simulink model "f8_VPP_demo_DER2"  (R2019b)
settings: Solver=VariableStepAuto  StartTime=0.0  StopTime=2  RelTol=1e-3
PreLoadFcn:
  | sr=0;ss=1;
InitFcn:
  | sr=0;ss=1;
undefined symbols (not defined in the file): Ion, Lithium
libraries: powerlib x185, powerlib_meascontrol x45, electricdrivelib x3, re_lib x3
(part 1 of 2)
settings Model: Creator=MAHMUD  LastModifiedBy=MAHMUD

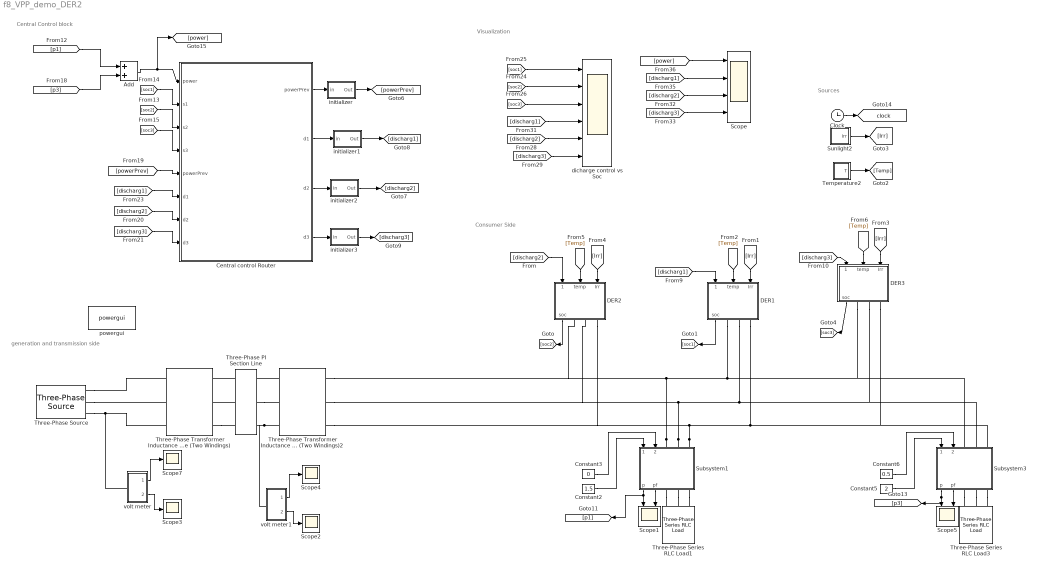
== system f8_VPP_demo_DER2 ==
  note: Consumer Side
  note: generation and transmission side
  note: Central Control block
  note: Visualization
  note: Sources
  Add : Sum  Inputs=2
  Central control Router : MATLAB Function  TreatAsAtomicUnit=on
  Clock : Clock
  Constant2 : Constant  Value=1.5
  Constant3 : Constant  Value=0
  Constant5 : Constant  Value=2
  Constant6 : Constant  Value=0.5
  DER1 : Subsystem
  DER2 : Subsystem
  DER3 : Subsystem
  Scope : Scope  NumInputPorts=4
  Scope1 : Scope  NumInputPorts=2
  Scope{2..4,7} (4 alike) : Scope
  Scope5 : Scope  NumInputPorts=2
  Subsystem1 : Subsystem
  Subsystem3 : Subsystem
  Sunlight2 : Subsystem
  Temperature2 : Subsystem
  Three-Phase PI Section Line : powerlib/Elements/Three-Phase PI Section Line  LConnTagsString=a|b|c  RConnTagsString=A|B|C  Frequency=50  Resistances=[ 0.01273 0.3864]  Inductances="[ 0.9337e-3  4.1264e-3]"  Capacitances=[12.74e-9 7.751e-9]  Length=100
      settings: SourceProductName=Simscape Electrical
  Three-Phase Series RLC Load1 : powerlib/Elements/Three-Phase Series RLC Load  LConnTagsString=A|B|C  Configuration=Y (grounded)  NominalVoltage=240  Vabc=[240 240 240]  Vabcp=[1e3 1e3 1e3]  NominalFrequency=50  UnbalancedPower=off  ActivePower=5e3  InductivePower=0  CapacitivePower=0  Pabc=[10e3 9e3 11e3]  QLabc=[100 90 110]  QCabc=[100 90 110]  Pabcp=[10e3 9e3 11e3]  QLabcp=[100 90 110]  QCabcp=[100 90 110]  Measurements=None  LoadType=constant PQ
      settings: SourceProductName=Simscape Electrical
  Three-Phase Series RLC Load3 : powerlib/Elements/Three-Phase Series RLC Load  LConnTagsString=A|B|C  Configuration=Y (grounded)  NominalVoltage=240  Vabc=[1e3 1e3 1e3]  Vabcp=[1e3 1e3 1e3]  NominalFrequency=50  UnbalancedPower=off  ActivePower=2e3  InductivePower=5e3  CapacitivePower=0  Pabc=[10e3 9e3 11e3]  QLabc=[100 90 110]  QCabc=[100 90 110]  Pabcp=[10e3 9e3 11e3]  QLabcp=[100 90 110]  QCabcp=[100 90 110]  Measurements=None  LoadType=constant PQ
      settings: SourceProductName=Simscape Electrical
  Three-Phase Source : powerlib/Electrical Sources/Three-Phase Source  InternalConnection=Yg  VoltagePhases=off  Voltage=14270  PhaseAngle=0  Voltage_phases=[25e3 25e3 25e3]/sqrt(3)  PhaseAngles_phases=[0 -120 +120]  Frequency=50  NonIdealSource=on  SpecifyImpedance=off  Resistance=0.8929  Inductance=0  ShortCircuitLevel=100e6  BaseVoltage=15000  XRratio=7  BusType=PQ  Pref=30e3  Qref=0  Prefabc=[10e3, 10e3, 10e3]  Qrefabc=[0, 0, 0]  Qmin=-inf  Qmax=inf
      settings: SourceProductName=Simscape Electrical
  Three-Phase Transformer Inductance Matrix Type (Two Windings) : powerlib/Elements/Three-Phase Transformer Inductance Matrix Type (Two Windings)  CoreType=Three-limb or five-limb core  Winding1Connection=Yg  Winding2Connection=Yg  AutoTransformer=off  Measurements=None  NominalPower=[100e3, 50]  VLLnom=[25000, 130000]  WindingResistances=[0.01, 0.01]  NoLoadIexcPos=2  NoLoadPlossPos=1000  ShortCircuitReactancePos=0.06  ShortCircuitReactancePosAuto=0.06  NoLoadIexcZero=100  NoLoadPlossZero=1500  ShortCircuitReactanceZero=0.03  ShortCircuitReactanceZeroAuto=0.03
      settings: SourceProductName=Simscape Electrical  SourceProductBaseCode=PS
  Three-Phase Transformer Inductance Matrix Type (Two Windings)2 : powerlib/Elements/Three-Phase Transformer Inductance Matrix Type (Two Windings)  CoreType=Three-limb or five-limb core  Winding1Connection=Yg  Winding2Connection=Yg  AutoTransformer=off  Measurements=None  NominalPower=[30e3, 50]  VLLnom=[12700, 240]  WindingResistances=[0.01, 0.01]  NoLoadIexcPos=4  NoLoadPlossPos=1000  ShortCircuitReactancePos=0.06  ShortCircuitReactancePosAuto=0.06  NoLoadIexcZero=100  NoLoadPlossZero=1500  ShortCircuitReactanceZero=0.03  ShortCircuitReactanceZeroAuto=0.03
      settings: SourceProductName=Simscape Electrical  SourceProductBaseCode=PS
  dicharge control vs Soc : Scope  NumInputPorts=6
  initializer : Subsystem
  initializer1 : Subsystem
  initializer2 : Subsystem
  initializer3 : Subsystem
  powergui : powerlib/powergui  Priority=1  SimulationMode=Continuous  SampleTime=50e-6  frequency=60  Iterations=50  frequencyindice=0  Pbase=100e6  ErrMax=1e-4  UnitsV=kV  UnitsW=MW  buscounter=0  FunctionMessages=off  echomessages=off  EnableUseOfTLC=off  CurrentSourceSwitches=off  DisableSnubberDevices=off  DisableRonSwitches=off  DisableVfSwitches=off  DisplayEquations=off  AutomaticDiscreteSolvers=off  SolverType=Tustin/Backward Euler (TBE)  Interpol=off  ExternalGateDelay=off  methode=off  Ts=100  x0status=blocks  SPID=on  SwTol=0  HookPort=off  NonlinearTolerance=1e-4  nMaxIteration=100  ContinueOnMaxIteration=off  RestoreLinks=warning  ResistiveCurrentMeasurement=off  Frange=[0:2:500]  Ylog=off  Xlog=on  ShowGrid=off  save=off  variable=ZData  structure=0  ZoomFFT=off  StartTime=0.0  cycles=1  DisplayStyle=1  fundamental=60  FreqAxis=off  MaxFrequency=1000  frequencyindicesteady=1  RmsSteady=1  display=off
      settings: SourceProductName=Simscape Electrical
  volt meter : Subsystem
  volt meter1 : Subsystem
  tag scope: clock=global
  wires:
  volt meter/1(Vsin) -> Scope7/1
  volt meter/2(Vrms) -> Scope3/1
  volt meter1/2(Vrms) -> Scope2/1
  volt meter1/1(Vsin) -> Scope4/1
  Subsystem1/1(p) -> [p1], Scope1/1
  Constant3/1 -> Subsystem1/2(start time)
  Constant6/1 -> Subsystem3/2(start time)
  Subsystem1/2(pf) -> Scope1/2
  Constant5/1 -> Subsystem3/1(stop time)
  Subsystem3/2(pf) -> Scope5/2
  Subsystem3/1(p) -> [p3], Scope5/1
  Constant2/1 -> Subsystem1/1(stop time)
  Temperature2/1(T) -> [Temp]
  Sunlight2/1(Irr) -> [Irr]
  [discharg2] -> DER2/1(discharging)
  [Temp] -> DER2/2(temp)
  [Irr] -> DER2/3(Irr)
  [Irr] -> DER1/3(Irr)
  [Temp] -> DER1/2(temp)
  [discharg1] -> DER1/1(discharging)
  [discharg3] -> DER3/1(discharging)
  [Temp] -> DER3/2(temp)
  [Irr] -> DER3/3(Irr)
  DER2/1(soc) -> [soc2]
  DER1/1(soc) -> [soc1]
  DER3/1(soc) -> [soc3]
  [p1] -> Add/1
  [p3] -> Add/2
  Central control Router/1(powerPrev) -> initializer/1(in)
  Central control Router/2(d1) -> initializer1/1(in)
  Central control Router/3(d2) -> initializer2/1(in)
  Central control Router/4(d3) -> initializer3/1(in)
  Add/1 -> [power], Central control Router/1(power)
  [soc3] -> Central control Router/4(s3)
  [soc1] -> Central control Router/2(s1)
  [soc2] -> Central control Router/3(s2)
  initializer3/1(Out) -> [discharg3]
  [powerPrev] -> Central control Router/5("powerPrev ")
  initializer/1(Out) -> [powerPrev]
  initializer2/1(Out) -> [discharg2]
  initializer1/1(Out) -> [discharg1]
  [discharg2] -> Central control Router/7("d2 ")
  [discharg3] -> Central control Router/8("d3 ")
  [discharg1] -> Central control Router/6("d1 ")
  Clock/1 -> [clock]
  [soc1] -> dicharge control vs Soc/1
  [soc2] -> dicharge control vs Soc/2
  [soc3] -> dicharge control vs Soc/3
  [power] -> Scope/1
  [discharg1] -> Scope/2
  [discharg2] -> Scope/3
  [discharg3] -> Scope/4
  [discharg1] -> dicharge control vs Soc/4
  [discharg2] -> dicharge control vs Soc/5
  [discharg3] -> dicharge control vs Soc/6
  connections:
  Three-Phase PI Section Line/RConn3 -- volt meter1/LConn1 -- Three-Phase Transformer Inductance Matrix Type (Two Windings)2/LConn3
  Three-Phase PI Section Line/RConn2 -- Three-Phase Transformer Inductance Matrix Type (Two Windings)2/LConn2
  Three-Phase PI Section Line/LConn1 -- Three-Phase Transformer Inductance Matrix Type (Two Windings)/RConn1
  Three-Phase Transformer Inductance Matrix Type (Two Windings)/RConn3 -- Three-Phase PI Section Line/LConn3
  Three-Phase PI Section Line/LConn2 -- Three-Phase Transformer Inductance Matrix Type (Two Windings)/RConn2
  Three-Phase Transformer Inductance Matrix Type (Two Windings)2/LConn1 -- Three-Phase PI Section Line/RConn1
  Three-Phase Source/RConn3 -- volt meter/LConn1 -- Three-Phase Transformer Inductance Matrix Type (Two Windings)/LConn3
  Three-Phase Source/RConn2 -- Three-Phase Transformer Inductance Matrix Type (Two Windings)/LConn2
  Three-Phase Source/RConn1 -- Three-Phase Transformer Inductance Matrix Type (Two Windings)/LConn1
  Subsystem1/LConn2 -- DER2/RConn2 -- Three-Phase Transformer Inductance Matrix Type (Two Windings)2/RConn2 -- Subsystem3/LConn2 -- DER3/RConn2 -- DER1/RConn2
  Subsystem1/LConn3 -- DER2/RConn3 -- Three-Phase Transformer Inductance Matrix Type (Two Windings)2/RConn3 -- Subsystem3/LConn3 -- DER3/RConn3 -- DER1/RConn3
  Subsystem1/LConn1 -- DER2/RConn1 -- Three-Phase Transformer Inductance Matrix Type (Two Windings)2/RConn1 -- Subsystem3/LConn1 -- DER3/RConn1 -- DER1/RConn1
  Subsystem1/RConn2 -- Three-Phase Series RLC Load1/LConn2
  Subsystem3/RConn3 -- Three-Phase Series RLC Load3/LConn3
  Subsystem3/RConn1 -- Three-Phase Series RLC Load3/LConn1
  Subsystem1/RConn1 -- Three-Phase Series RLC Load1/LConn1
  Subsystem1/RConn3 -- Three-Phase Series RLC Load1/LConn3
  Subsystem3/RConn2 -- Three-Phase Series RLC Load3/LConn2

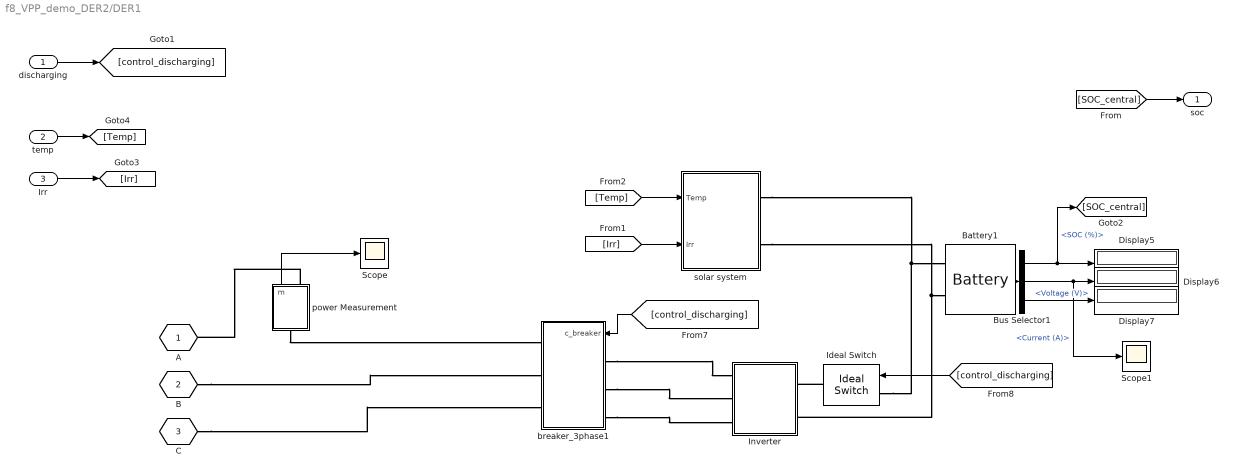
== system f8_VPP_demo_DER2/DER1 ==
  discharging : Inport
  temp : Inport  Port=2
  Irr : Inport  Port=3
  Battery1 : electricdrivelib/Extra Sources/Battery  BatType=Lithium-Ion  ShowTempParam=off  ThermalPreset=no  ShowAgeParam=off  NomV=100  NomQ=1000  SOC=5  Batt_Tr=0.1  PresetModel=on  MaxQ=1000  MinV=75  FullV=116.3987  Dis_rate=434.7826  R=0.001  Normal_OP=904.3478  expZone="[108.0386      49.13043]"  current=[6.5 13 32.5]  Units=Time  Tci=20  NomT=20  T2=-30  MaxQ2=4.8  FullV2=7.1  Normal_OP2=5.655  expZone2="[6.58           1]"  Rca=0.6  ti=2000  Dp=0  Neq0=0  Tsim=1e6  Ta1=25  Qeol=5.4*0.9  Reol=0.013333*1.2  Char_age=[2.3478, 3]  Dis_age=[2.3478, 10]  N1=1500  N2=10500  N3=1000  N4=1400  Ta2=45  N5=950
  Bus Selector1 : BusSelector  OutputSignals=SOC (%),Current (A),Voltage (V)
  Display5 : Display
  Display6 : Display
  Display7 : Display
  Ideal Switch : powerlib/Power Electronics/Ideal Switch  Ron=0.001  Lon=0  IC=0  Rs=1e5  Cs=inf  Measurements=off
      settings: SourceProductName=Simscape Electrical
  Inverter : Subsystem
  Scope : Scope
  Scope1 : Scope
  breaker_3phase1 : Subsystem
  power Measurement : Subsystem
  "solar system " : Subsystem
  A : PMIOPort  Tag=PMCPort  Side=Right
  B : PMIOPort  Tag=PMCPort  Port=2  Side=Right
  C : PMIOPort  Tag=PMCPort  Port=3  Side=Right
  soc : Outport
  wires:
  [SOC_central] -> soc/1
  [Temp] -> "solar system "/1(Temp)
  [Irr] -> "solar system "/2(Irr)
  temp/1 -> [Temp]
  Irr/1 -> [Irr]
  discharging/1 -> [control_discharging]
  [control_discharging] -> breaker_3phase1/1(c_breaker)
  [control_discharging] -> Ideal Switch/1
  power Measurement/1(m) -> Scope/1
  Bus Selector1/1 -> Display5/1, [SOC_central]  "<SOC (%)>"
  Battery1/1 -> Bus Selector1/1
  Bus Selector1/3 -> Display7/1  "<Voltage (V)>"
  Bus Selector1/2 -> Display6/1, Scope1/1  "<Current (A)>"
  connections:
  power Measurement/LConn1 -- breaker_3phase1/RConn1
  B/RConn1 -- breaker_3phase1/RConn2
  C/RConn1 -- breaker_3phase1/RConn3
  power Measurement/RConn1 -- A/RConn1
  breaker_3phase1/LConn2 -- Inverter/RConn2
  breaker_3phase1/LConn3 -- Inverter/RConn3
  breaker_3phase1/LConn1 -- Inverter/RConn1
  Ideal Switch/RConn1 -- Inverter/LConn1
  Battery1/LConn2 -- Inverter/LConn2 -- "solar system "/RConn2
  "solar system "/RConn1 -- Ideal Switch/LConn1 -- Battery1/LConn1

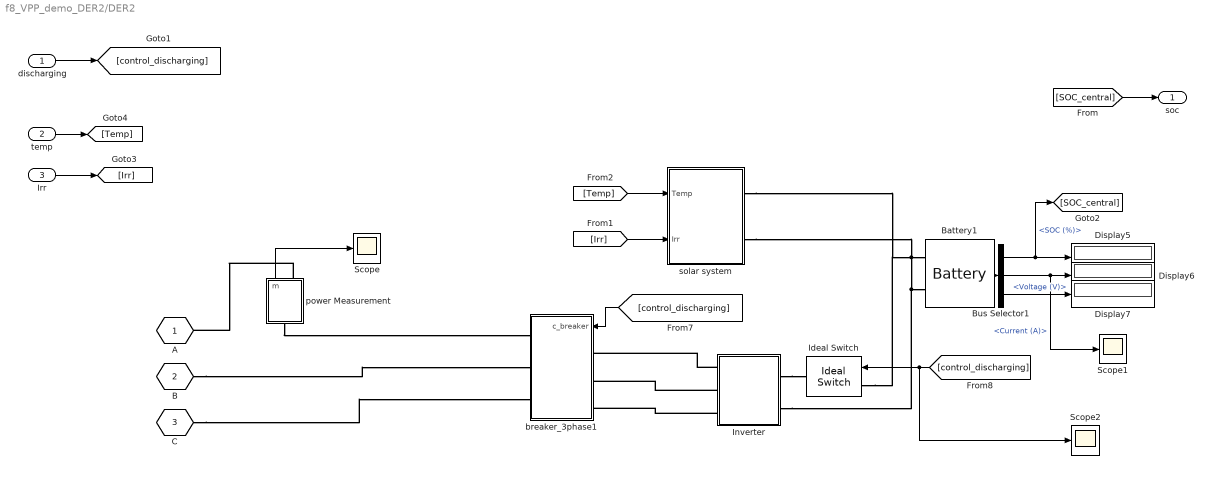
== system f8_VPP_demo_DER2/DER2 ==
  discharging : Inport
  temp : Inport  Port=2
  Irr : Inport  Port=3
  Battery1 : electricdrivelib/Extra Sources/Battery  BatType=Lithium-Ion  ShowTempParam=off  ThermalPreset=no  ShowAgeParam=off  NomV=100  NomQ=1000  SOC=50  Batt_Tr=0.1  PresetModel=on  MaxQ=1000  MinV=75  FullV=116.3987  Dis_rate=434.7826  R=0.001  Normal_OP=904.3478  expZone="[108.0386      49.13043]"  current=[6.5 13 32.5]  Units=Time  Tci=20  NomT=20  T2=-30  MaxQ2=4.8  FullV2=7.1  Normal_OP2=5.655  expZone2="[6.58           1]"  Rca=0.6  ti=2000  Dp=0  Neq0=0  Tsim=1e6  Ta1=25  Qeol=5.4*0.9  Reol=0.013333*1.2  Char_age=[2.3478, 3]  Dis_age=[2.3478, 10]  N1=1500  N2=10500  N3=1000  N4=1400  Ta2=45  N5=950
  Bus Selector1 : BusSelector  OutputSignals=SOC (%),Current (A),Voltage (V)
  Display5 : Display
  Display6 : Display
  Display7 : Display
  Ideal Switch : powerlib/Power Electronics/Ideal Switch  Ron=0.001  Lon=0  IC=0  Rs=1e5  Cs=inf  Measurements=off
      settings: SourceProductName=Simscape Electrical
  Inverter : Subsystem
  Scope : Scope
  Scope1 : Scope
  Scope2 : Scope
  breaker_3phase1 : Subsystem
  power Measurement : Subsystem
  "solar system " : Subsystem
  A : PMIOPort  Tag=PMCPort  Side=Right
  B : PMIOPort  Tag=PMCPort  Port=2  Side=Right
  C : PMIOPort  Tag=PMCPort  Port=3  Side=Right
  soc : Outport
  wires:
  Bus Selector1/2 -> Scope1/1, Display6/1  "<Current (A)>"
  Bus Selector1/3 -> Display7/1  "<Voltage (V)>"
  Battery1/1 -> Bus Selector1/1
  Bus Selector1/1 -> [SOC_central], Display5/1  "<SOC (%)>"
  power Measurement/1(m) -> Scope/1
  [control_discharging] -> Scope2/1, Ideal Switch/1
  [control_discharging] -> breaker_3phase1/1(c_breaker)
  discharging/1 -> [control_discharging]
  Irr/1 -> [Irr]
  temp/1 -> [Temp]
  [Irr] -> "solar system "/2(Irr)
  [Temp] -> "solar system "/1(Temp)
  [SOC_central] -> soc/1
  connections:
  Battery1/LConn1 -- Ideal Switch/LConn1 -- "solar system "/RConn1
  "solar system "/RConn2 -- Inverter/LConn2 -- Battery1/LConn2
  Inverter/LConn1 -- Ideal Switch/RConn1
  Inverter/RConn1 -- breaker_3phase1/LConn1
  Inverter/RConn3 -- breaker_3phase1/LConn3
  Inverter/RConn2 -- breaker_3phase1/LConn2
  power Measurement/RConn1 -- A/RConn1
  C/RConn1 -- breaker_3phase1/RConn3
  B/RConn1 -- breaker_3phase1/RConn2
  power Measurement/LConn1 -- breaker_3phase1/RConn1

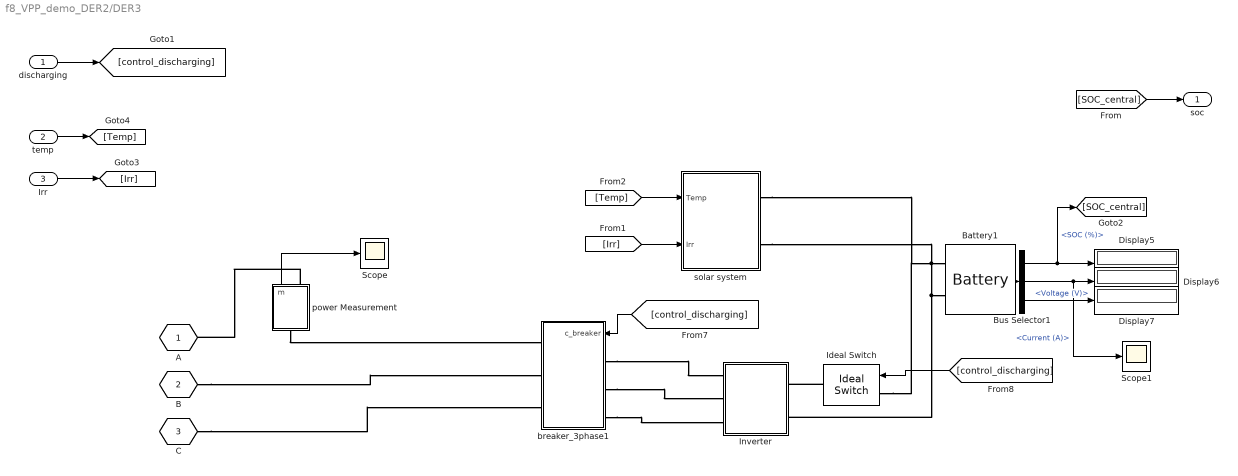
== system f8_VPP_demo_DER2/DER3 ==
  discharging : Inport
  temp : Inport  Port=2
  Irr : Inport  Port=3
  Battery1 : electricdrivelib/Extra Sources/Battery  BatType=Lithium-Ion  ShowTempParam=off  ThermalPreset=no  ShowAgeParam=off  NomV=100  NomQ=1000  SOC=90  Batt_Tr=0.1  PresetModel=on  MaxQ=1000  MinV=75  FullV=116.3987  Dis_rate=434.7826  R=0.001  Normal_OP=904.3478  expZone="[108.0386      49.13043]"  current=[6.5 13 32.5]  Units=Time  Tci=20  NomT=20  T2=-30  MaxQ2=4.8  FullV2=7.1  Normal_OP2=5.655  expZone2="[6.58           1]"  Rca=0.6  ti=2000  Dp=0  Neq0=0  Tsim=1e6  Ta1=25  Qeol=5.4*0.9  Reol=0.013333*1.2  Char_age=[2.3478, 3]  Dis_age=[2.3478, 10]  N1=1500  N2=10500  N3=1000  N4=1400  Ta2=45  N5=950
  Bus Selector1 : BusSelector  OutputSignals=SOC (%),Current (A),Voltage (V)
  Display5 : Display
  Display6 : Display
  Display7 : Display
  Ideal Switch : powerlib/Power Electronics/Ideal Switch  Ron=0.001  Lon=0  IC=0  Rs=1e5  Cs=inf  Measurements=off
      settings: SourceProductName=Simscape Electrical
  Inverter : Subsystem
  Scope : Scope
  Scope1 : Scope
  breaker_3phase1 : Subsystem
  power Measurement : Subsystem
  "solar system " : Subsystem
  A : PMIOPort  Tag=PMCPort  Side=Right
  B : PMIOPort  Tag=PMCPort  Port=2  Side=Right
  C : PMIOPort  Tag=PMCPort  Port=3  Side=Right
  soc : Outport
  wires:
  Bus Selector1/2 -> Scope1/1, Display6/1  "<Current (A)>"
  Bus Selector1/3 -> Display7/1  "<Voltage (V)>"
  Battery1/1 -> Bus Selector1/1
  Bus Selector1/1 -> [SOC_central], Display5/1  "<SOC (%)>"
  power Measurement/1(m) -> Scope/1
  [control_discharging] -> Ideal Switch/1
  [control_discharging] -> breaker_3phase1/1(c_breaker)
  discharging/1 -> [control_discharging]
  Irr/1 -> [Irr]
  temp/1 -> [Temp]
  [Irr] -> "solar system "/2(Irr)
  [Temp] -> "solar system "/1(Temp)
  [SOC_central] -> soc/1
  connections:
  Battery1/LConn1 -- Ideal Switch/LConn1 -- "solar system "/RConn1
  "solar system "/RConn2 -- Inverter/LConn2 -- Battery1/LConn2
  Ideal Switch/RConn1 -- Inverter/LConn1
  breaker_3phase1/LConn1 -- Inverter/RConn1
  breaker_3phase1/LConn3 -- Inverter/RConn3
  breaker_3phase1/LConn2 -- Inverter/RConn2
  power Measurement/RConn1 -- A/RConn1
  C/RConn1 -- breaker_3phase1/RConn3
  B/RConn1 -- breaker_3phase1/RConn2
  power Measurement/LConn1 -- breaker_3phase1/RConn1

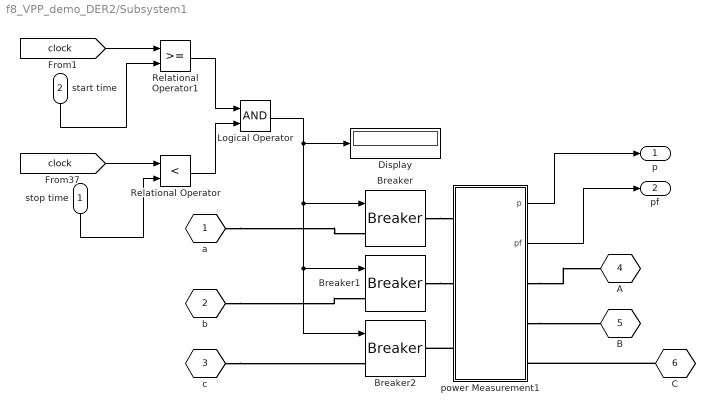
== system f8_VPP_demo_DER2/Subsystem1 ==
  stop time : Inport
  start time : Inport  Port=2
  Breaker : powerlib/Elements/Breaker  InitialState=0  SwitchingTimes="[1/60  5/60]"  External=on  BreakerResistance=0.01  SnubberResistance=1e6  SnubberCapacitance=inf  Measurements=None  MoreParameters=on  NoBreakLoop=off
      settings: SourceProductName=Simscape Electrical
  Breaker1 : powerlib/Elements/Breaker  InitialState=0  SwitchingTimes="[1/60  5/60]"  External=on  BreakerResistance=0.01  SnubberResistance=1e6  SnubberCapacitance=inf  Measurements=None  MoreParameters=on  NoBreakLoop=off
      settings: SourceProductName=Simscape Electrical
  Breaker2 : powerlib/Elements/Breaker  InitialState=0  SwitchingTimes="[1/60  5/60]"  External=on  BreakerResistance=0.01  SnubberResistance=1e6  SnubberCapacitance=inf  Measurements=None  MoreParameters=on  NoBreakLoop=off
      settings: SourceProductName=Simscape Electrical
  Display : Display
  Logical Operator : Logic  AllPortsSameDT=off  OutDataTypeStr=boolean
  Relational Operator : RelationalOperator  Operator=<  OutDataTypeStr=boolean  ZeroCross=off  RndMeth=Simplest
  Relational Operator1 : RelationalOperator  OutDataTypeStr=boolean  ZeroCross=off  RndMeth=Simplest
  power Measurement1 : Subsystem
  a : PMIOPort  Tag=PMCPort  Side=Left
  b : PMIOPort  Tag=PMCPort  Port=2  Side=Left
  c : PMIOPort  Tag=PMCPort  Port=3  Side=Left
  "A " : PMIOPort  Tag=PMCPort  Port=4  Side=Right
  B : PMIOPort  Tag=PMCPort  Port=5  Side=Right
  C : PMIOPort  Tag=PMCPort  Port=6  Side=Right
  p : Outport
  pf : Outport  Port=2
  wires:
  Logical Operator/1 -> Breaker/1, Breaker2/1, Breaker1/1, Display/1
  [clock] -> Relational Operator/1
  stop time/1 -> Relational Operator/2
  [clock] -> Relational Operator1/1
  start time/1 -> Relational Operator1/2
  Relational Operator1/1 -> Logical Operator/1
  Relational Operator/1 -> Logical Operator/2
  power Measurement1/2(pf) -> pf/1
  power Measurement1/1(p) -> p/1
  connections:
  b/RConn1 -- Breaker1/LConn1
  c/RConn1 -- Breaker2/LConn1
  a/RConn1 -- Breaker/LConn1
  power Measurement1/RConn2 -- B/RConn1
  power Measurement1/LConn3 -- Breaker2/RConn1
  Breaker1/RConn1 -- power Measurement1/LConn2
  Breaker/RConn1 -- power Measurement1/LConn1
  C/RConn1 -- power Measurement1/RConn3
  power Measurement1/RConn1 -- "A "/RConn1

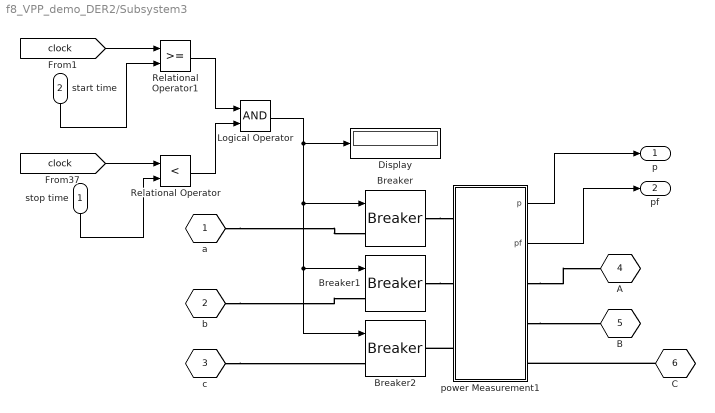
== system f8_VPP_demo_DER2/Subsystem3 ==
  stop time : Inport
  start time : Inport  Port=2
  Breaker : powerlib/Elements/Breaker  InitialState=0  SwitchingTimes="[1/60  5/60]"  External=on  BreakerResistance=0.01  SnubberResistance=1e6  SnubberCapacitance=inf  Measurements=None  MoreParameters=on  NoBreakLoop=off
      settings: SourceProductName=Simscape Electrical
  Breaker1 : powerlib/Elements/Breaker  InitialState=0  SwitchingTimes="[1/60  5/60]"  External=on  BreakerResistance=0.01  SnubberResistance=1e6  SnubberCapacitance=inf  Measurements=None  MoreParameters=on  NoBreakLoop=off
      settings: SourceProductName=Simscape Electrical
  Breaker2 : powerlib/Elements/Breaker  InitialState=0  SwitchingTimes="[1/60  5/60]"  External=on  BreakerResistance=0.01  SnubberResistance=1e6  SnubberCapacitance=inf  Measurements=None  MoreParameters=on  NoBreakLoop=off
      settings: SourceProductName=Simscape Electrical
  Display : Display
  Logical Operator : Logic  AllPortsSameDT=off  OutDataTypeStr=boolean
  Relational Operator : RelationalOperator  Operator=<  OutDataTypeStr=boolean  ZeroCross=off  RndMeth=Simplest
  Relational Operator1 : RelationalOperator  OutDataTypeStr=boolean  ZeroCross=off  RndMeth=Simplest
  power Measurement1 : Subsystem
  a : PMIOPort  Tag=PMCPort  Side=Left
  b : PMIOPort  Tag=PMCPort  Port=2  Side=Left
  c : PMIOPort  Tag=PMCPort  Port=3  Side=Left
  "A " : PMIOPort  Tag=PMCPort  Port=4  Side=Right
  B : PMIOPort  Tag=PMCPort  Port=5  Side=Right
  C : PMIOPort  Tag=PMCPort  Port=6  Side=Right
  p : Outport
  pf : Outport  Port=2
  wires:
  Logical Operator/1 -> Breaker/1, Breaker2/1, Breaker1/1, Display/1
  [clock] -> Relational Operator/1
  stop time/1 -> Relational Operator/2
  [clock] -> Relational Operator1/1
  start time/1 -> Relational Operator1/2
  Relational Operator1/1 -> Logical Operator/1
  Relational Operator/1 -> Logical Operator/2
  power Measurement1/2(pf) -> pf/1
  power Measurement1/1(p) -> p/1
  connections:
  b/RConn1 -- Breaker1/LConn1
  c/RConn1 -- Breaker2/LConn1
  a/RConn1 -- Breaker/LConn1
  power Measurement1/RConn2 -- B/RConn1
  power Measurement1/LConn3 -- Breaker2/RConn1
  Breaker1/RConn1 -- power Measurement1/LConn2
  Breaker/RConn1 -- power Measurement1/LConn1
  C/RConn1 -- power Measurement1/RConn3
  power Measurement1/RConn1 -- "A "/RConn1

== system f8_VPP_demo_DER2/Sunlight2 ==
  Constant4 : Constant  Value=ss
  Logical Operator : Logic  Operator=NOT  AllPortsSameDT=off  OutDataTypeStr=boolean
  Product : Product
  Relational Operator : RelationalOperator  OutDataTypeStr=boolean  ZeroCross=off  RndMeth=Simplest
  Sine Wave Function : Sin  Amplitude=500  Frequency=3.14*(ss-sr)  SampleTime=0  VectorParams1D=off
  Irr : Outport
  wires:
  Product/1 -> Irr/1
  Constant4/1 -> Relational Operator/2
  Logical Operator/1 -> Product/2
  [clock] -> Relational Operator/1
  Relational Operator/1 -> Logical Operator/1
  Sine Wave Function/1 -> Product/1

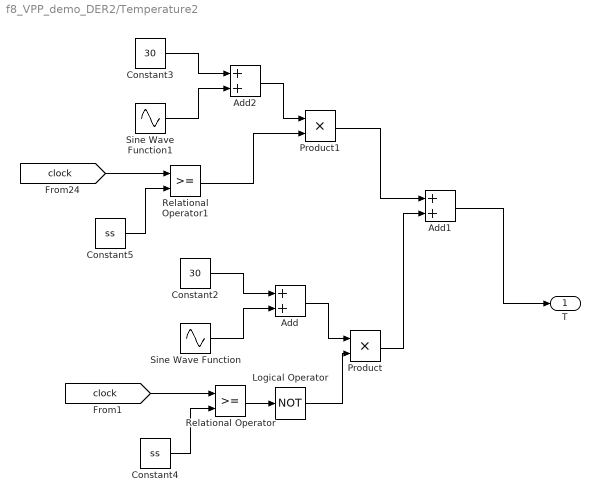
== system f8_VPP_demo_DER2/Temperature2 ==
  Add : Sum
  Add1 : Sum
  Add2 : Sum
  Constant2 : Constant  Value=30
  Constant3 : Constant  Value=30
  Constant4 : Constant  Value=ss
  Constant5 : Constant  Value=ss
  Logical Operator : Logic  Operator=NOT  AllPortsSameDT=off  OutDataTypeStr=boolean
  Product : Product
  Product1 : Product
  Relational Operator : RelationalOperator  OutDataTypeStr=boolean  ZeroCross=off  RndMeth=Simplest
  Relational Operator1 : RelationalOperator  OutDataTypeStr=boolean  ZeroCross=off  RndMeth=Simplest
  Sine Wave Function : Sin  Amplitude=5  Frequency=3.14*(ss-sr)  SampleTime=0  VectorParams1D=off
  Sine Wave Function1 : Sin  Amplitude=3  Frequency=3.14*(ss-sr)  SampleTime=0  VectorParams1D=off
  T : Outport
  wires:
  Constant4/1 -> Relational Operator/2
  [clock] -> Relational Operator/1
  Relational Operator1/1 -> Product1/2
  Constant2/1 -> Add/1
  Add2/1 -> Product1/1
  Constant3/1 -> Add2/1
  Logical Operator/1 -> Product/2
  Product1/1 -> Add1/1
  Constant5/1 -> Relational Operator1/2
  Sine Wave Function/1 -> Add/2
  Sine Wave Function1/1 -> Add2/2
  Product/1 -> Add1/2
  Relational Operator/1 -> Logical Operator/1
  Add1/1 -> T/1
  Add/1 -> Product/1
  [clock] -> Relational Operator1/1

== system f8_VPP_demo_DER2/initializer ==
  in : Inport
  Constant5 : Constant  Value=0
  Switch : Switch  Criteria=u2 > Threshold  ZeroCross=off
  Out : Outport
  wires:
  Constant5/1 -> Switch/3
  [clock] -> Switch/2
  in/1 -> Switch/1
  Switch/1 -> Out/1

== system f8_VPP_demo_DER2/initializer1 ==
  in : Inport
  Constant5 : Constant  Value=0
  Switch : Switch  Criteria=u2 > Threshold  ZeroCross=off
  Out : Outport
  wires:
  Switch/1 -> Out/1
  in/1 -> Switch/1
  [clock] -> Switch/2
  Constant5/1 -> Switch/3

== system f8_VPP_demo_DER2/initializer2 ==
  in : Inport
  Constant5 : Constant  Value=0
  Switch : Switch  Criteria=u2 > Threshold  ZeroCross=off
  Out : Outport
  wires:
  Constant5/1 -> Switch/3
  [clock] -> Switch/2
  in/1 -> Switch/1
  Switch/1 -> Out/1

== system f8_VPP_demo_DER2/initializer3 ==
  in : Inport
  Constant5 : Constant  Value=0
  Switch : Switch  Criteria=u2 > Threshold  ZeroCross=off
  Out : Outport
  wires:
  Switch/1 -> Out/1
  in/1 -> Switch/1
  [clock] -> Switch/2
  Constant5/1 -> Switch/3

== system f8_VPP_demo_DER2/volt meter ==
  First-Order Filter2 : powerlib_meascontrol/Filters/First-Order Filter  FilterType=Lowpass  Tc=100e-3  Ts=0  Initialize=off  Vac_Init=[0, 0, 50]  Vdc_Init=0  PlotResponse=off  FreqRange="[0,  200,  1]"
      settings: SourceProductName=Simscape Electrical
  Ground3 : powerlib/Elements/Ground  LConnTagsString=a
      settings: SourceProductName=Simscape Electrical
  RMS2 : powerlib_meascontrol/Measurements/RMS  TrueRMS=on  Freq=50  RMSInit=210  Ts=0.001
      settings: SourceProductName=Simscape Electrical
  Voltage Measurement3 : powerlib/Measurements/Voltage Measurement  PhasorSimulation=off  OutputType=Complex  PSBequivalent=0
      settings: SourceProductName=Simscape Electrical
  In : PMIOPort  Side=Left
  Vsin : Outport
  Vrms : Outport  Port=2
  wires:
  Voltage Measurement3/1 -> Vsin/1, RMS2/1
  RMS2/1 -> First-Order Filter2/1
  First-Order Filter2/1 -> Vrms/1
  connections:
  Ground3/LConn1 -- Voltage Measurement3/LConn2
  Voltage Measurement3/LConn1 -- In/RConn1

== system f8_VPP_demo_DER2/volt meter1 ==
  First-Order Filter2 : powerlib_meascontrol/Filters/First-Order Filter  FilterType=Lowpass  Tc=100e-3  Ts=0  Initialize=off  Vac_Init=[0, 0, 50]  Vdc_Init=0  PlotResponse=off  FreqRange="[0,  200,  1]"
      settings: SourceProductName=Simscape Electrical
  Ground3 : powerlib/Elements/Ground  LConnTagsString=a
      settings: SourceProductName=Simscape Electrical
  RMS2 : powerlib_meascontrol/Measurements/RMS  TrueRMS=on  Freq=50  RMSInit=210  Ts=0.001
      settings: SourceProductName=Simscape Electrical
  Voltage Measurement3 : powerlib/Measurements/Voltage Measurement  PhasorSimulation=off  OutputType=Complex  PSBequivalent=0
      settings: SourceProductName=Simscape Electrical
  In : PMIOPort  Side=Left
  Vsin : Outport
  Vrms : Outport  Port=2
  wires:
  First-Order Filter2/1 -> Vrms/1
  RMS2/1 -> First-Order Filter2/1
  Voltage Measurement3/1 -> RMS2/1, Vsin/1
  connections:
  Voltage Measurement3/LConn1 -- In/RConn1
  Ground3/LConn1 -- Voltage Measurement3/LConn2

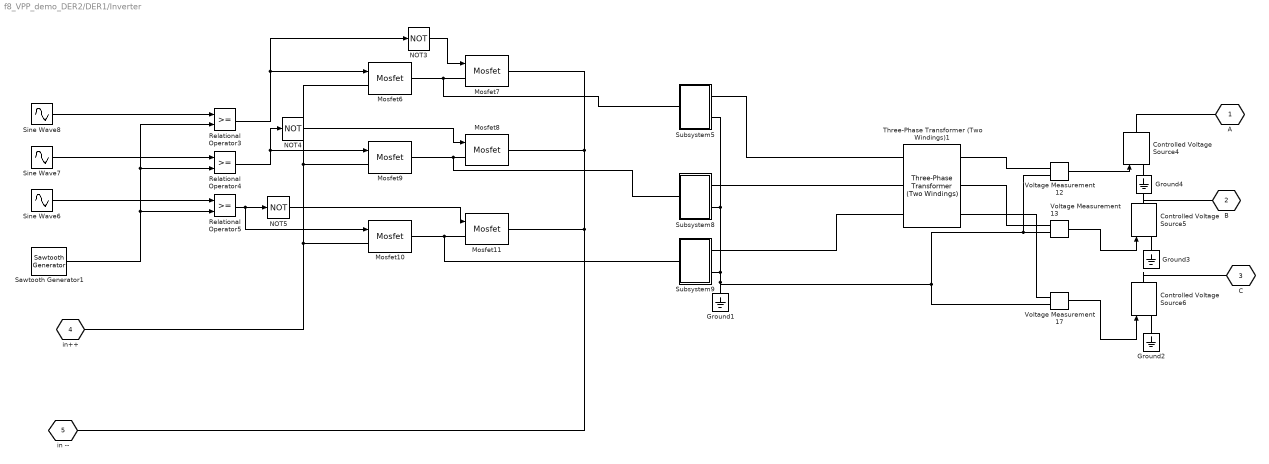
== system f8_VPP_demo_DER2/DER1/Inverter ==
  Controlled Voltage Source4 : powerlib/Electrical Sources/Controlled Voltage Source  Initialize=on  Source_Type=AC  Amplitude=0  Phase=0  Frequency=0  Measurements=None
      settings: SourceProductName=Simscape Electrical
  Controlled Voltage Source5 : powerlib/Electrical Sources/Controlled Voltage Source  Initialize=on  Source_Type=AC  Amplitude=0  Phase=0  Frequency=0  Measurements=None
      settings: SourceProductName=Simscape Electrical
  Controlled Voltage Source6 : powerlib/Electrical Sources/Controlled Voltage Source  Initialize=on  Source_Type=AC  Amplitude=0  Phase=0  Frequency=0  Measurements=None
      settings: SourceProductName=Simscape Electrical
  Ground{1..4} (4 alike) : powerlib/Elements/Ground  LConnTagsString=a
      settings: SourceProductName=Simscape Electrical
  Mosfet{6..11} (6 alike) : powerlib/Power Electronics/Mosfet  Ron=0.1  Lon=0  Rd=0.01  Vfd=0  IC=0  Rs=1e5  Cs=inf  Measurements=off
      settings: SourceProductName=Simscape Electrical
  NOT3 : Logic  Operator=NOT  IconShape=distinctive  AllPortsSameDT=off  OutDataTypeStr=boolean
  NOT4 : Logic  Operator=NOT  IconShape=distinctive  AllPortsSameDT=off  OutDataTypeStr=boolean
  NOT5 : Logic  Operator=NOT  IconShape=distinctive  AllPortsSameDT=off  OutDataTypeStr=boolean
  Relational Operator3 : RelationalOperator  OutDataTypeStr=boolean  ZeroCross=off  RndMeth=Simplest
  Relational Operator4 : RelationalOperator  OutDataTypeStr=boolean  ZeroCross=off  RndMeth=Simplest
  Relational Operator5 : RelationalOperator  OutDataTypeStr=boolean  ZeroCross=off  RndMeth=Simplest
  Sawtooth Generator1 : powerlib_meascontrol/Pulse & Signal Generators/Sawtooth Generator  Freq=1e3  Phase=180  Ts=0
      settings: SourceProductName=Simscape Electrical
  Sine Wave6 : Sin  Frequency=2*pi*50  Phase=4*pi/3  SampleTime=0
  Sine Wave7 : Sin  Frequency=2*pi*50  Phase=2*pi/3  SampleTime=0
  Sine Wave8 : Sin  Frequency=2*pi*50  SampleTime=0
  Subsystem5 : Subsystem
  Subsystem8 : Subsystem
  Subsystem9 : Subsystem
  Three-Phase Transformer (Two Windings)1 : powerlib/Elements/Three-Phase Transformer (Two Windings)  Winding1Connection=Yg  Winding2Connection=Yg  CoreType=Three single-phase transformers  SetSaturation=off  Hysteresis=off  DataFile='hysteresis'  SetInitialFlux=off  Measurements=None  UNITS=pu  NominalPower=[ 1e3 , 50 ]  Winding1=[ 31.5 , 0.002 , 0.08 ]  Winding2=[ 240 , 0.002 , 0.08 ]  Rm=500  Lm=500  L0=0.5  Saturation=[ 0,0 ; 0.0024,1.2 ; 1.0,1.52 ]  InitialFluxes=[ 0.8 , -0.8 , 0.7 ]  BreakLoop=off  DiscreteSolver=Trapezoidal iterative  DataType=off  TransfoNumber=1
      settings: SourceProductName=Simscape Electrical
  Voltage Measurement12 : powerlib/Measurements/Voltage Measurement  PhasorSimulation=off  OutputType=Complex  PSBequivalent=0
      settings: SourceProductName=Simscape Electrical
  Voltage Measurement13 : powerlib/Measurements/Voltage Measurement  PhasorSimulation=off  OutputType=Complex  PSBequivalent=0
      settings: SourceProductName=Simscape Electrical
  Voltage Measurement17 : powerlib/Measurements/Voltage Measurement  PhasorSimulation=off  OutputType=Complex  PSBequivalent=0
      settings: SourceProductName=Simscape Electrical
  A : PMIOPort  Tag=PMCPort  Side=Right
  B : PMIOPort  Tag=PMCPort  Port=2  Side=Right
  C : PMIOPort  Tag=PMCPort  Port=3  Side=Right
  in++ : PMIOPort  Tag=PMCPort  Port=4  Side=Left
  in -- : PMIOPort  Tag=PMCPort  Port=5  Side=Left
  wires:
  Voltage Measurement13/1 -> Controlled Voltage Source5/1
  NOT5/1 -> Mosfet11/1
  Voltage Measurement12/1 -> Controlled Voltage Source4/1
  Sine Wave6/1 -> Relational Operator5/1
  Sine Wave7/1 -> Relational Operator4/1
  Relational Operator4/1 -> Mosfet9/1, NOT4/1
  NOT4/1 -> Mosfet8/1
  Voltage Measurement17/1 -> Controlled Voltage Source6/1
  Sawtooth Generator1/1 -> Relational Operator3/2, Relational Operator4/2, Relational Operator5/2
  Sine Wave8/1 -> Relational Operator3/1
  NOT3/1 -> Mosfet7/1
  Relational Operator5/1 -> Mosfet10/1, NOT5/1
  Relational Operator3/1 -> NOT3/1, Mosfet6/1
  connections:
  Three-Phase Transformer (Two Windings)1/RConn1 -- Voltage Measurement12/LConn1
  Controlled Voltage Source6/RConn1 -- C/RConn1
  Controlled Voltage Source5/RConn1 -- B/RConn1
  Three-Phase Transformer (Two Windings)1/RConn3 -- Voltage Measurement17/LConn1
  Ground3/LConn1 -- Controlled Voltage Source5/LConn1
  Three-Phase Transformer (Two Windings)1/RConn2 -- Voltage Measurement13/LConn1
  Controlled Voltage Source4/RConn1 -- A/RConn1
  Ground2/LConn1 -- Controlled Voltage Source6/LConn1
  Ground4/LConn1 -- Controlled Voltage Source4/LConn1
  Mosfet10/LConn1 -- in++/RConn1 -- Mosfet9/LConn1 -- Mosfet6/LConn1
  Three-Phase Transformer (Two Windings)1/LConn3 -- Subsystem9/RConn1
  Mosfet9/RConn1 -- Mosfet8/LConn1 -- Subsystem8/LConn1
  Subsystem8/RConn1 -- Three-Phase Transformer (Two Windings)1/LConn2
  Mosfet11/LConn1 -- Mosfet10/RConn1 -- Subsystem9/LConn1
  Three-Phase Transformer (Two Windings)1/LConn1 -- Subsystem5/RConn1
  Mosfet6/RConn1 -- Mosfet7/LConn1 -- Subsystem5/LConn1
  Mosfet7/RConn1 -- Mosfet8/RConn1 -- in --/RConn1 -- Mosfet11/RConn1
  Subsystem9/RConn2 -- Voltage Measurement17/LConn2 -- Voltage Measurement13/LConn2 -- Voltage Measurement12/LConn2 -- Ground1/LConn1 -- Subsystem8/RConn2 -- Subsystem5/RConn2

== system f8_VPP_demo_DER2/DER1/breaker_3phase1 ==
  c_breaker : Inport
  Breaker : powerlib/Elements/Breaker  InitialState=0  SwitchingTimes="[1/60  5/60]"  External=on  BreakerResistance=0.01  SnubberResistance=1e6  SnubberCapacitance=inf  Measurements=None  MoreParameters=on  NoBreakLoop=off
      settings: SourceProductName=Simscape Electrical
  Breaker1 : powerlib/Elements/Breaker  InitialState=0  SwitchingTimes="[1/60  5/60]"  External=on  BreakerResistance=0.01  SnubberResistance=1e6  SnubberCapacitance=inf  Measurements=None  MoreParameters=on  NoBreakLoop=off
      settings: SourceProductName=Simscape Electrical
  Breaker2 : powerlib/Elements/Breaker  InitialState=0  SwitchingTimes="[1/60  5/60]"  External=on  BreakerResistance=0.01  SnubberResistance=1e6  SnubberCapacitance=inf  Measurements=None  MoreParameters=on  NoBreakLoop=off
      settings: SourceProductName=Simscape Electrical
  a : PMIOPort  Tag=PMCPort  Side=Right
  A : PMIOPort  Tag=PMCPort  Port=2  Side=Left
  B : PMIOPort  Tag=PMCPort  Port=3  Side=Left
  C : PMIOPort  Tag=PMCPort  Port=4  Side=Left
  b : PMIOPort  Tag=PMCPort  Port=5  Side=Right
  c : PMIOPort  Tag=PMCPort  Port=6  Side=Right
  wires:
  c_breaker/1 -> Breaker/1, Breaker2/1, Breaker1/1
  connections:
  C/RConn1 -- Breaker2/LConn1
  b/RConn1 -- Breaker1/RConn1
  a/RConn1 -- Breaker/RConn1
  c/RConn1 -- Breaker2/RConn1
  A/RConn1 -- Breaker/LConn1
  B/RConn1 -- Breaker1/LConn1

== system f8_VPP_demo_DER2/DER1/power Measurement ==
  Current Measurement1 : powerlib/Measurements/Current Measurement  PhasorSimulation=off  OutputType=Complex  PSBequivalent=0
      settings: SourceProductName=Simscape Electrical
  First-Order Filter : powerlib_meascontrol/Filters/First-Order Filter  FilterType=Lowpass  Tc=100e-3  Ts=0  Initialize=off  Vac_Init=[0, 0, 50]  Vdc_Init=0  PlotResponse=off  FreqRange="[0,  200,  1]"
      settings: SourceProductName=Simscape Electrical
  First-Order Filter1 : powerlib_meascontrol/Filters/First-Order Filter  FilterType=Lowpass  Tc=100e-3  Ts=0  Initialize=off  Vac_Init=[0, 0, 50]  Vdc_Init=0  PlotResponse=off  FreqRange="[0,  200,  1]"
      settings: SourceProductName=Simscape Electrical
  Gain : Gain  Gain=3
  Ground1 : powerlib/Elements/Ground  LConnTagsString=a
      settings: SourceProductName=Simscape Electrical
  Product : Product
  RMS : powerlib_meascontrol/Measurements/RMS  TrueRMS=on  Freq=50  RMSInit=210  Ts=0.001
      settings: SourceProductName=Simscape Electrical
  RMS1 : powerlib_meascontrol/Measurements/RMS  TrueRMS=on  Freq=50  RMSInit=210  Ts=0.001
      settings: SourceProductName=Simscape Electrical
  Scope{,1..3} (4 alike) : Scope
  Voltage Measurement1 : powerlib/Measurements/Voltage Measurement  PhasorSimulation=off  OutputType=Complex  PSBequivalent=0
      settings: SourceProductName=Simscape Electrical
  "out " : PMIOPort  Tag=PMCPort  Side=Right
  in : PMIOPort  Tag=PMCPort  Port=2  Side=Left
  m : Outport
  wires:
  Product/1 -> Gain/1
  First-Order Filter/1 -> Product/2, Scope3/1
  First-Order Filter1/1 -> Scope2/1, Product/1
  Voltage Measurement1/1 -> RMS/1, Scope/1
  RMS1/1 -> First-Order Filter1/1
  RMS/1 -> First-Order Filter/1
  Gain/1 -> m/1
  Current Measurement1/1 -> RMS1/1, Scope1/1
  connections:
  "out "/RConn1 -- Current Measurement1/RConn1
  Voltage Measurement1/LConn1 -- in/RConn1 -- Current Measurement1/LConn1
  Ground1/LConn1 -- Voltage Measurement1/LConn2

== system f8_VPP_demo_DER2/DER1/solar system  ==
  Temp : Inport
  Irr : Inport  Port=2
  Bus Selector : BusSelector  OutputSignals=V_PV
  Current Measurement1 : powerlib/Measurements/Current Measurement  PhasorSimulation=off  OutputType=Complex  PSBequivalent=0
  PV Array : re_lib/Solar/PV Array  Npar=40  Nser=10  PlotType=array @ 1000 W/m2 & specified temperatures  S_vec="[ 1000  500  100 ]"  Temp_C_vec="[ 45 25  ]"  ModuleName=1Soltech 1STH-215-P  PlotWhenSelected=off  Pm=213.15  Ncell=60  Voc=36.3  Isc=7.84  Vm=29  Im=7.35  beta_Voc_pc=-0.36099  alpha_Isc_pc=0.102  beta_Voc=-0.13104  alpha_Isc=0.007997  IL=7.8649  I0=2.9259e-10  nI=0.98117  Rsh=313.3991  Rs=0.39383  BAL=off  Tc=1e-6  Tfilter=5e-5
      settings: SourceProductName=Simscape Electrical
  Scope2 : Scope
  Scope3 : Scope
  Series RLC Branch1 : powerlib/Elements/Series RLC Branch  LConnTagsString=__new0  RConnTagsString=__new0  BranchType=R  Resistance=1000000  Inductance=1e-3  SetiL0=off  InitialCurrent=0  Capacitance=1e-6  Setx0=off  InitialVoltage=0  Measurements=None
      settings: SourceProductName=Simscape Electrical
  baterry ++ : PMIOPort  Tag=PMCPort  Side=Right
  baterry -- : PMIOPort  Tag=PMCPort  Port=2  Side=Right
  wires:
  Bus Selector/1 -> Scope2/1  "<V_PV>"
  PV Array/1 -> Bus Selector/1
  Irr/1 -> PV Array/1
  Temp/1 -> PV Array/2
  Current Measurement1/1 -> Scope3/1
  connections:
  Series RLC Branch1/LConn1 -- Current Measurement1/LConn1 -- PV Array/RConn1
  Current Measurement1/RConn1 -- baterry ++/RConn1
  Series RLC Branch1/RConn1 -- baterry --/RConn1 -- PV Array/RConn2

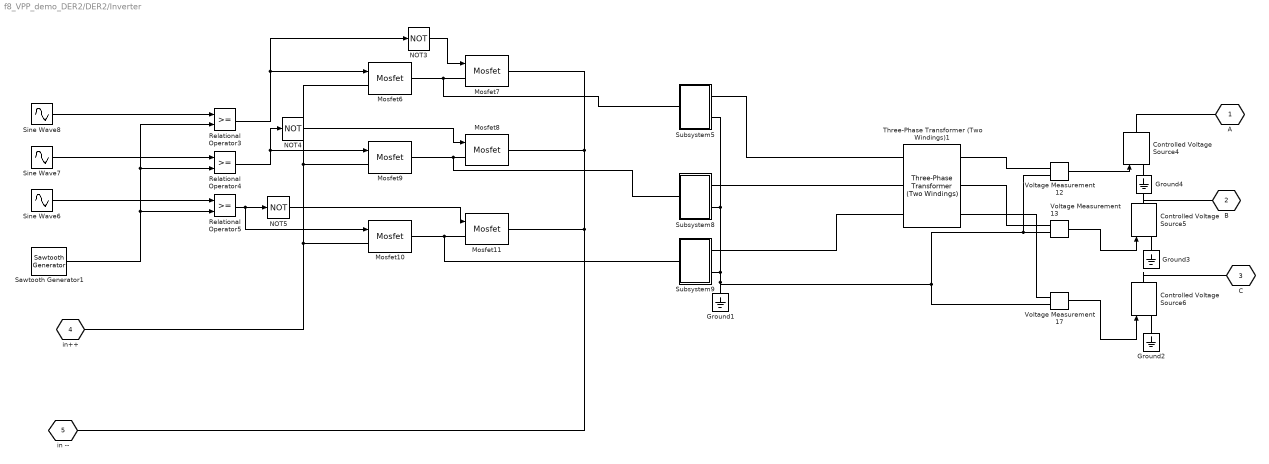
== system f8_VPP_demo_DER2/DER2/Inverter ==
  Controlled Voltage Source4 : powerlib/Electrical Sources/Controlled Voltage Source  Initialize=on  Source_Type=AC  Amplitude=0  Phase=0  Frequency=0  Measurements=None
      settings: SourceProductName=Simscape Electrical
  Controlled Voltage Source5 : powerlib/Electrical Sources/Controlled Voltage Source  Initialize=on  Source_Type=AC  Amplitude=0  Phase=0  Frequency=0  Measurements=None
      settings: SourceProductName=Simscape Electrical
  Controlled Voltage Source6 : powerlib/Electrical Sources/Controlled Voltage Source  Initialize=on  Source_Type=AC  Amplitude=0  Phase=0  Frequency=0  Measurements=None
      settings: SourceProductName=Simscape Electrical
  Ground{1..4} (4 alike) : powerlib/Elements/Ground  LConnTagsString=a
      settings: SourceProductName=Simscape Electrical
  Mosfet{6..11} (6 alike) : powerlib/Power Electronics/Mosfet  Ron=0.1  Lon=0  Rd=0.01  Vfd=0  IC=0  Rs=1e5  Cs=inf  Measurements=off
      settings: SourceProductName=Simscape Electrical
  NOT3 : Logic  Operator=NOT  IconShape=distinctive  AllPortsSameDT=off  OutDataTypeStr=boolean
  NOT4 : Logic  Operator=NOT  IconShape=distinctive  AllPortsSameDT=off  OutDataTypeStr=boolean
  NOT5 : Logic  Operator=NOT  IconShape=distinctive  AllPortsSameDT=off  OutDataTypeStr=boolean
  Relational Operator3 : RelationalOperator  OutDataTypeStr=boolean  ZeroCross=off  RndMeth=Simplest
  Relational Operator4 : RelationalOperator  OutDataTypeStr=boolean  ZeroCross=off  RndMeth=Simplest
  Relational Operator5 : RelationalOperator  OutDataTypeStr=boolean  ZeroCross=off  RndMeth=Simplest
  Sawtooth Generator1 : powerlib_meascontrol/Pulse & Signal Generators/Sawtooth Generator  Freq=1e3  Phase=180  Ts=0
      settings: SourceProductName=Simscape Electrical
  Sine Wave6 : Sin  Frequency=2*pi*50  Phase=4*pi/3  SampleTime=0
  Sine Wave7 : Sin  Frequency=2*pi*50  Phase=2*pi/3  SampleTime=0
  Sine Wave8 : Sin  Frequency=2*pi*50  SampleTime=0
  Subsystem5 : Subsystem
  Subsystem8 : Subsystem
  Subsystem9 : Subsystem
  Three-Phase Transformer (Two Windings)1 : powerlib/Elements/Three-Phase Transformer (Two Windings)  Winding1Connection=Yg  Winding2Connection=Yg  CoreType=Three single-phase transformers  SetSaturation=off  Hysteresis=off  DataFile='hysteresis'  SetInitialFlux=off  Measurements=None  UNITS=pu  NominalPower=[ 1e3 , 50 ]  Winding1=[ 31.5 , 0.002 , 0.08 ]  Winding2=[ 240 , 0.002 , 0.08 ]  Rm=500  Lm=500  L0=0.5  Saturation=[ 0,0 ; 0.0024,1.2 ; 1.0,1.52 ]  InitialFluxes=[ 0.8 , -0.8 , 0.7 ]  BreakLoop=off  DiscreteSolver=Trapezoidal iterative  DataType=off  TransfoNumber=1
      settings: SourceProductName=Simscape Electrical
  Voltage Measurement12 : powerlib/Measurements/Voltage Measurement  PhasorSimulation=off  OutputType=Complex  PSBequivalent=0
      settings: SourceProductName=Simscape Electrical
  Voltage Measurement13 : powerlib/Measurements/Voltage Measurement  PhasorSimulation=off  OutputType=Complex  PSBequivalent=0
      settings: SourceProductName=Simscape Electrical
  Voltage Measurement17 : powerlib/Measurements/Voltage Measurement  PhasorSimulation=off  OutputType=Complex  PSBequivalent=0
      settings: SourceProductName=Simscape Electrical
  A : PMIOPort  Tag=PMCPort  Side=Right
  B : PMIOPort  Tag=PMCPort  Port=2  Side=Right
  C : PMIOPort  Tag=PMCPort  Port=3  Side=Right
  in++ : PMIOPort  Tag=PMCPort  Port=4  Side=Left
  in -- : PMIOPort  Tag=PMCPort  Port=5  Side=Left
  wires:
  Voltage Measurement13/1 -> Controlled Voltage Source5/1
  NOT5/1 -> Mosfet11/1
  Voltage Measurement12/1 -> Controlled Voltage Source4/1
  Sine Wave6/1 -> Relational Operator5/1
  Sine Wave7/1 -> Relational Operator4/1
  Relational Operator4/1 -> Mosfet9/1, NOT4/1
  NOT4/1 -> Mosfet8/1
  Voltage Measurement17/1 -> Controlled Voltage Source6/1
  Sawtooth Generator1/1 -> Relational Operator3/2, Relational Operator4/2, Relational Operator5/2
  Sine Wave8/1 -> Relational Operator3/1
  NOT3/1 -> Mosfet7/1
  Relational Operator5/1 -> Mosfet10/1, NOT5/1
  Relational Operator3/1 -> NOT3/1, Mosfet6/1
  connections:
  Three-Phase Transformer (Two Windings)1/RConn1 -- Voltage Measurement12/LConn1
  Controlled Voltage Source6/RConn1 -- C/RConn1
  Controlled Voltage Source5/RConn1 -- B/RConn1
  Three-Phase Transformer (Two Windings)1/RConn3 -- Voltage Measurement17/LConn1
  Ground3/LConn1 -- Controlled Voltage Source5/LConn1
  Three-Phase Transformer (Two Windings)1/RConn2 -- Voltage Measurement13/LConn1
  Controlled Voltage Source4/RConn1 -- A/RConn1
  Ground2/LConn1 -- Controlled Voltage Source6/LConn1
  Ground4/LConn1 -- Controlled Voltage Source4/LConn1
  Mosfet10/LConn1 -- in++/RConn1 -- Mosfet9/LConn1 -- Mosfet6/LConn1
  Three-Phase Transformer (Two Windings)1/LConn3 -- Subsystem9/RConn1
  Mosfet9/RConn1 -- Mosfet8/LConn1 -- Subsystem8/LConn1
  Subsystem8/RConn1 -- Three-Phase Transformer (Two Windings)1/LConn2
  Mosfet11/LConn1 -- Mosfet10/RConn1 -- Subsystem9/LConn1
  Three-Phase Transformer (Two Windings)1/LConn1 -- Subsystem5/RConn1
  Mosfet6/RConn1 -- Mosfet7/LConn1 -- Subsystem5/LConn1
  Mosfet7/RConn1 -- Mosfet8/RConn1 -- in --/RConn1 -- Mosfet11/RConn1
  Subsystem9/RConn2 -- Voltage Measurement17/LConn2 -- Voltage Measurement13/LConn2 -- Voltage Measurement12/LConn2 -- Ground1/LConn1 -- Subsystem8/RConn2 -- Subsystem5/RConn2

== system f8_VPP_demo_DER2/DER2/breaker_3phase1 ==
  c_breaker : Inport
  Breaker : powerlib/Elements/Breaker  InitialState=0  SwitchingTimes="[1/60  5/60]"  External=on  BreakerResistance=0.01  SnubberResistance=1e6  SnubberCapacitance=inf  Measurements=None  MoreParameters=on  NoBreakLoop=off
      settings: SourceProductName=Simscape Electrical
  Breaker1 : powerlib/Elements/Breaker  InitialState=0  SwitchingTimes="[1/60  5/60]"  External=on  BreakerResistance=0.01  SnubberResistance=1e6  SnubberCapacitance=inf  Measurements=None  MoreParameters=on  NoBreakLoop=off
      settings: SourceProductName=Simscape Electrical
  Breaker2 : powerlib/Elements/Breaker  InitialState=0  SwitchingTimes="[1/60  5/60]"  External=on  BreakerResistance=0.01  SnubberResistance=1e6  SnubberCapacitance=inf  Measurements=None  MoreParameters=on  NoBreakLoop=off
      settings: SourceProductName=Simscape Electrical
  a : PMIOPort  Tag=PMCPort  Side=Right
  A : PMIOPort  Tag=PMCPort  Port=2  Side=Left
  B : PMIOPort  Tag=PMCPort  Port=3  Side=Left
  C : PMIOPort  Tag=PMCPort  Port=4  Side=Left
  b : PMIOPort  Tag=PMCPort  Port=5  Side=Right
  c : PMIOPort  Tag=PMCPort  Port=6  Side=Right
  wires:
  c_breaker/1 -> Breaker1/1, Breaker2/1, Breaker/1
  connections:
  B/RConn1 -- Breaker1/LConn1
  A/RConn1 -- Breaker/LConn1
  c/RConn1 -- Breaker2/RConn1
  a/RConn1 -- Breaker/RConn1
  b/RConn1 -- Breaker1/RConn1
  C/RConn1 -- Breaker2/LConn1

== system f8_VPP_demo_DER2/DER2/power Measurement ==
  Current Measurement1 : powerlib/Measurements/Current Measurement  PhasorSimulation=off  OutputType=Complex  PSBequivalent=0
      settings: SourceProductName=Simscape Electrical
  First-Order Filter : powerlib_meascontrol/Filters/First-Order Filter  FilterType=Lowpass  Tc=100e-3  Ts=0  Initialize=off  Vac_Init=[0, 0, 50]  Vdc_Init=0  PlotResponse=off  FreqRange="[0,  200,  1]"
      settings: SourceProductName=Simscape Electrical
  First-Order Filter1 : powerlib_meascontrol/Filters/First-Order Filter  FilterType=Lowpass  Tc=100e-3  Ts=0  Initialize=off  Vac_Init=[0, 0, 50]  Vdc_Init=0  PlotResponse=off  FreqRange="[0,  200,  1]"
      settings: SourceProductName=Simscape Electrical
  Gain : Gain  Gain=3
  Ground1 : powerlib/Elements/Ground  LConnTagsString=a
      settings: SourceProductName=Simscape Electrical
  Product : Product
  RMS : powerlib_meascontrol/Measurements/RMS  TrueRMS=on  Freq=50  RMSInit=210  Ts=0.001
      settings: SourceProductName=Simscape Electrical
  RMS1 : powerlib_meascontrol/Measurements/RMS  TrueRMS=on  Freq=50  RMSInit=210  Ts=0.001
      settings: SourceProductName=Simscape Electrical
  Scope{,1..3} (4 alike) : Scope
  Voltage Measurement1 : powerlib/Measurements/Voltage Measurement  PhasorSimulation=off  OutputType=Complex  PSBequivalent=0
      settings: SourceProductName=Simscape Electrical
  "out " : PMIOPort  Tag=PMCPort  Side=Right
  in : PMIOPort  Tag=PMCPort  Port=2  Side=Left
  m : Outport
  wires:
  Current Measurement1/1 -> Scope1/1, RMS1/1
  Gain/1 -> m/1
  RMS/1 -> First-Order Filter/1
  RMS1/1 -> First-Order Filter1/1
  Voltage Measurement1/1 -> Scope/1, RMS/1
  First-Order Filter1/1 -> Product/1, Scope2/1
  First-Order Filter/1 -> Scope3/1, Product/2
  Product/1 -> Gain/1
  connections:
  Ground1/LConn1 -- Voltage Measurement1/LConn2
  Current Measurement1/LConn1 -- in/RConn1 -- Voltage Measurement1/LConn1
  "out "/RConn1 -- Current Measurement1/RConn1

== system f8_VPP_demo_DER2/DER2/solar system  ==
  Temp : Inport
  Irr : Inport  Port=2
  Bus Selector : BusSelector  OutputSignals=V_PV
  Current Measurement1 : powerlib/Measurements/Current Measurement  PhasorSimulation=off  OutputType=Complex  PSBequivalent=0
  PV Array : re_lib/Solar/PV Array  Npar=40  Nser=10  PlotType=array @ 1000 W/m2 & specified temperatures  S_vec="[ 1000  500  100 ]"  Temp_C_vec="[ 45 25  ]"  ModuleName=1Soltech 1STH-215-P  PlotWhenSelected=off  Pm=213.15  Ncell=60  Voc=36.3  Isc=7.84  Vm=29  Im=7.35  beta_Voc_pc=-0.36099  alpha_Isc_pc=0.102  beta_Voc=-0.13104  alpha_Isc=0.007997  IL=7.8649  I0=2.9259e-10  nI=0.98117  Rsh=313.3991  Rs=0.39383  BAL=off  Tc=1e-6  Tfilter=5e-5
      settings: SourceProductName=Simscape Electrical
  Scope2 : Scope
  Scope3 : Scope
  Series RLC Branch1 : powerlib/Elements/Series RLC Branch  LConnTagsString=__new0  RConnTagsString=__new0  BranchType=R  Resistance=1000000  Inductance=1e-3  SetiL0=off  InitialCurrent=0  Capacitance=1e-6  Setx0=off  InitialVoltage=0  Measurements=None
      settings: SourceProductName=Simscape Electrical
  baterry ++ : PMIOPort  Tag=PMCPort  Side=Right
  baterry -- : PMIOPort  Tag=PMCPort  Port=2  Side=Right
  wires:
  Current Measurement1/1 -> Scope3/1
  Temp/1 -> PV Array/2
  Irr/1 -> PV Array/1
  PV Array/1 -> Bus Selector/1
  Bus Selector/1 -> Scope2/1  "<V_PV>"
  connections:
  PV Array/RConn2 -- baterry --/RConn1 -- Series RLC Branch1/RConn1
  Current Measurement1/RConn1 -- baterry ++/RConn1
  PV Array/RConn1 -- Current Measurement1/LConn1 -- Series RLC Branch1/LConn1
